simulink model "system7"  (R2019a)
settings: Solver=ode45  StartTime=0.0  StopTime=stop_time  FixedStep=0.05  RelTol=1e-3
values from neighbouring files (symbols this model uses):
  b = 0    [Lab2.m]
settings Model: Creator=Vasco  LastModifiedBy=Vasco

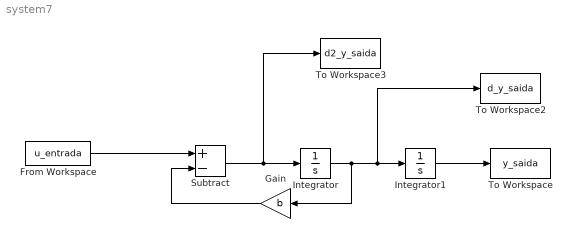
== system system7 ==
  From Workspace : FromWorkspace  VariableName=u_entrada  SampleTime=0
  Gain : Gain  Gain=b
  Integrator : Integrator
  Integrator1 : Integrator  InitialCondition=1
  Subtract : Sum  Inputs=+-
  To Workspace : ToWorkspace  VariableName=y_saida  SampleTime=-1
      settings: Save2DSignal=2-D array (concatenate along first dimension)
  To Workspace2 : ToWorkspace  VariableName=d_y_saida  SampleTime=-1
      settings: Save2DSignal=2-D array (concatenate along first dimension)
  To Workspace3 : ToWorkspace  VariableName=d2_y_saida  SampleTime=-1
      settings: Save2DSignal=2-D array (concatenate along first dimension)
  wires:
  From Workspace/1 -> Subtract/1
  Subtract/1 -> To Workspace3/1, Integrator/1
  Integrator/1 -> Gain/1, To Workspace2/1, Integrator1/1
  Integrator1/1 -> To Workspace/1
  Gain/1 -> Subtract/2
